simulink model "TankProgram"  (R2015a)
settings: Solver=ode45  StartTime=0.0  StopTime=10.0  RelTol=1e-3
settings Model: Creator=apaciull  LastModifiedBy=greg
settings DebuggingCC: UnderspecifiedInitializationDetection=Classic  MergeDetectMultiDrivingBlocksExec=none  SolverPrmCheckMsg=warning  StateNameClashWarn=warning

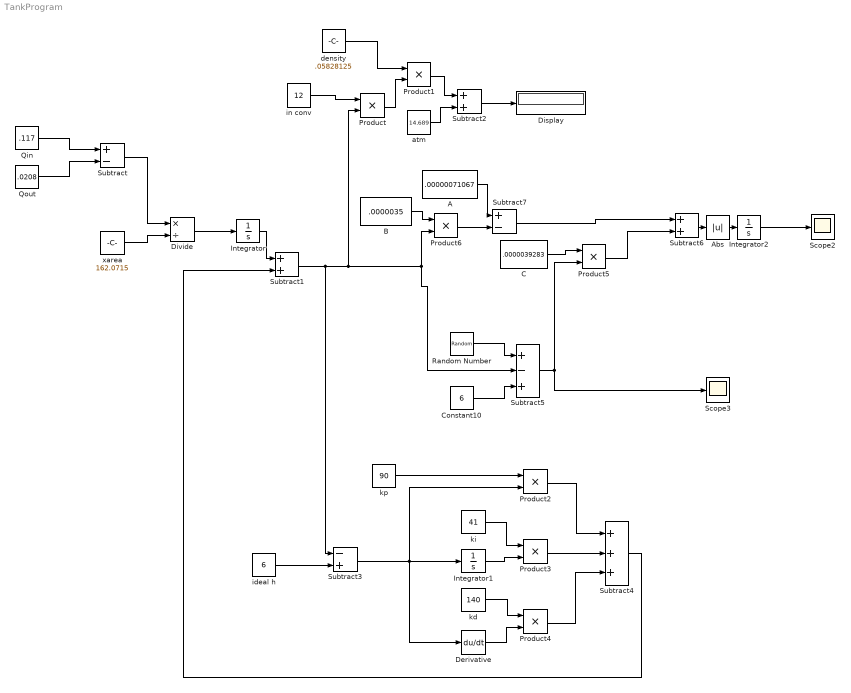
== system TankProgram ==
  A : Constant  Value=.00000071067
  Abs : Abs
  B : Constant  Value=.0000035
  C : Constant  Value=.0000039283
  Constant10 : Constant  Value=6
  Derivative : Derivative
  Display : Display
  Divide : Product  Inputs=*/
  Integrator : Integrator
  Integrator1 : Integrator
  Integrator2 : Integrator
  Product{,1..6} (7 alike) : Product
  Qin : Constant  Value=.117
  Qout : Constant  Value=.0208
  Random Number : RandomNumber  Variance=2  SampleTime=0.1
  Scope2 : Scope
      settings: SaveName=ScopeData2
  Scope3 : Scope
      settings: SaveName=ScopeData3
  Subtract : Sum  Inputs=+-
  Subtract1 : Sum
  Subtract2 : Sum
  Subtract3 : Sum  Inputs=-+
  Subtract4 : Sum  Inputs=+++
  Subtract5 : Sum  Inputs=+-+
  Subtract6 : Sum
  Subtract7 : Sum  Inputs=+-
  atm : Constant  Value=14.689
  density : Constant  Value=.05828125
  ideal h : Constant  Value=6
  in conv : Constant  Value=12
  kd : Constant  Value=140
  ki : Constant  Value=41
  kp : Constant  Value=90
  xarea : Constant  Value=162.0715
  wires:
  Qin/1 -> Subtract/1
  Qout/1 -> Subtract/2
  Subtract/1 -> Divide/1
  xarea/1 -> Divide/2
  Divide/1 -> Integrator/1
  Integrator/1 -> Subtract1/1
  Subtract1/1 -> Subtract5/2, Product6/2, Product/2, Subtract3/1
  in conv/1 -> Product/1
  density/1 -> Product1/1
  Product/1 -> Product1/2
  Product1/1 -> Subtract2/1
  atm/1 -> Subtract2/2
  Subtract2/1 -> Display/1
  ideal h/1 -> Subtract3/2
  Subtract3/1 -> Product2/2, Derivative/1, Integrator1/1
  kp/1 -> Product2/1
  ki/1 -> Product3/1
  Integrator1/1 -> Product3/2
  kd/1 -> Product4/1
  Derivative/1 -> Product4/2
  Product2/1 -> Subtract4/1
  Product3/1 -> Subtract4/2
  Product4/1 -> Subtract4/3
  Subtract4/1 -> Subtract1/2
  Constant10/1 -> Subtract5/3
  Subtract5/1 -> Scope3/1, Product5/2
  C/1 -> Product5/1
  Subtract6/1 -> Abs/1
  Integrator2/1 -> Scope2/1
  B/1 -> Product6/1
  Product6/1 -> Subtract7/2
  A/1 -> Subtract7/1
  Subtract7/1 -> Subtract6/1
  Product5/1 -> Subtract6/2
  Random Number/1 -> Subtract5/1
  Abs/1 -> Integrator2/1
